simulink model "M1_ASE_be_SE"  (R2022b)
settings: Solver=ode4  StartTime=0.0  StopTime=200  FixedStep=1e-3  RelTol=1e-3  AbsTol=1e-3  EnableMultiTasking=on
values from neighbouring files (symbols this model uses):
  BAT = TWIZ.BAT    [init_M1_ASE_be_SE_main.m]
  CHAS = TWIZ.CHAS    [init_M1_ASE_be_SE_main.m]
  COR = TWIZ.COR    [init_M1_ASE_be_SE_main.m]
  ENV = TWIZ.ENV    [init_M1_ASE_be_SE_main.m]
  HACH = TWIZ.HACH    [init_M1_ASE_be_SE_main.m]
  MCC = TWIZ.MCC    [init_M1_ASE_be_SE_main.m]
  TRANS = TWIZ.TRANS    [init_M1_ASE_be_SE_main.m]
libraries: simulink x1
settings Model: Creator=Walter  LastModifiedBy=WENPAGNAGDE_JUSTIN
settings SolverCC: AutoScaleAbsTol=off  AlgebraicLoopSolver=TrustRegion
settings DataIOCC: LimitDataPoints=on  SaveFormat=Array  SignalLoggingSaveFormat=ModelDataLogs  ReturnWorkspaceOutputs=off
settings OptimizationCC: ExpressionDepthLimit=2147483647  InitFltsAndDblsToZero=on  LifeSpan=inf
settings DebuggingCC: UnderspecifiedInitializationDetection=Classic  MergeDetectMultiDrivingBlocksExec=none  SolverPrmCheckMsg=warning  FcnCallInpInsideContextMsg=warning  UnconnectedInputMsg=warning  UnconnectedOutputMsg=warning  UnconnectedLineMsg=warning  StateNameClashWarn=warning  SFUnexpectedBacktrackingDiag=warning  SFNoUnconditionalDefaultTransitionDiag=warning  SFExecutionAtInitializationDiag=none  SFMachineParentedDataDiag=warning  ArithmeticOperatorsInVariantConditions=warning
settings HardwareCC: ProdBitPerPointer=32  ProdBitPerSizeT=32  ProdBitPerPtrDiffT=32  ProdLargestAtomicFloat=None  ProdIntDivRoundTo=Undefined  ProdEndianess=Unspecified  ProdWordSize=32  ProdHWDeviceType=32-bit Generic
settings ModelReferenceCC: EnableRefExpFcnMdlSchedulingChecks=on  PropagateSignalLabelsOutOfModel=off
settings SFSimCC: SimUseLocalCustomCode=off  CustomCodeUndefinedFunction=UseInterfaceOnly
settings RTWCC: RTWUseLocalCustomCode=off  DLArmComputeVersion=19.05
settings CodeAppCC: StateflowObjectComments=on
settings GRTTargetCC: TargetLangStandard=C89/C90 (ANSI)  CombineOutputUpdateFcns=off  GRTInterface=on
settings ConfigComp: CovMetricSettings=dw  CovSaveCumulativeToWorkspaceVar=on  CovSaveSingleToWorkspaceVar=on

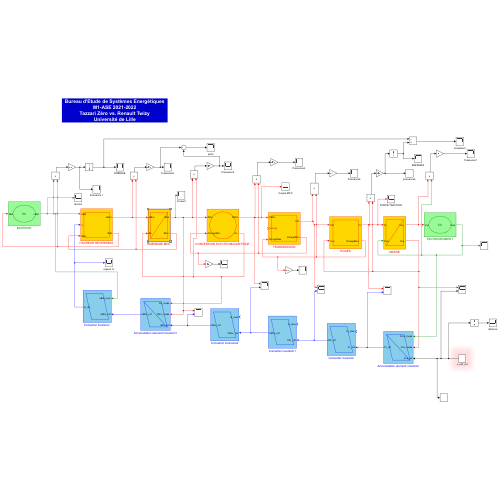
[thumbnail: Simulink's stored preview of the top-level diagram]
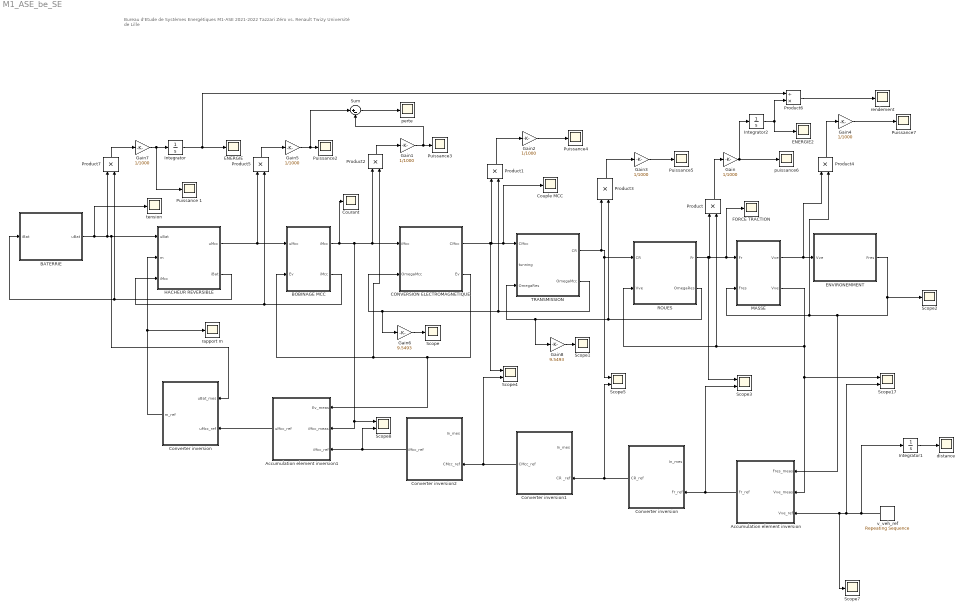
== system M1_ASE_be_SE ==
  note: Bureau d'Etude de Systèmes Energétiques
      | M1-ASE 2021-2022
      | Tazzari Zéro vs. Renault Twizy
      | Université de Lille
  Accumulation element inversion : Subsystem  AncestorBlock=simulink/SMC/Asservissement Correcteur IP
      settings: LibrarySourceBlock=|
      | simulink/SMC/Asservissement
      | Correcteur IP
      mask Display: plot(0,0,100,100, [10,30,90,70,10,90],[90,10,10,90,90,10])
  Accumulation element inversion1 : Subsystem  AncestorBlock=simulink/SMC/Asservissement Correcteur IP
      settings: LibrarySourceBlock=|
      | simulink/SMC/Asservissement
      | Correcteur IP
      mask Display: plot(0,0,100,100, [10,30,90,70,10,90],[90,10,10,90,90,10])
  BATERRIE : Subsystem  AncestorBlock=simulink/REM/SE
      settings: LibrarySourceBlock=simulink/REM/SE
      mask Display:
      | plot(0,0,100,100, 1.2*[50,57.68,60.77,63.08,64.97,66.58,68,69.26,70.4, 	71.42,72.36,78.28,80,78.28,72.36,71.42,70.4, 	69.26,68,66.58,64.97,63.08,60.77,57.68,50,42.32, 	39.23,36.92,35.03,33.42,32,30.74,29.6,28.58, 	27.64,21.72,20,21.72,27.64,28.58,29.6,30.74,32, 	33.42,35.03,36.92,39.23,42.32,50]-10, 1.2*[20,21,22,23,24,25,26,27,28,29,30,40,50,60,70,71,72, 	73,74,75,76,77,78,79,80,79,78,77,76,75,74,73,72, 	71,70,60,50,40,30,29,28,27,26,25,24,23,22,21,20]-10)
      | disp('ES')
  BOBINAGE MCC : Subsystem  AncestorBlock=simulink/REM/EA  mask(CM){}
      settings: LibrarySourceBlock=simulink/REM/EA
      mask Display: plot(0,0,100,100,[10,10,90,90,10],[90,10,10,90,90], [10,90],[10,90])
  "CONVERSION ELECTROMAGNETIQUE " : Subsystem  AncestorBlock=simulink/REM/EC EM
      settings: LibrarySourceBlock=simulink/REM/EC EM
      mask Display: plot(0,0,100,100, 1.4*[50,57.68,60.77,63.08,64.97,66.58,68,69.26,70.4, 	71.42,72.36,78.28,80,78.28,72.36,71.42,70.4, 	69.26,68,66.58,64.97,63.08,60.77,57.68,50,42.32, 	39.23,36.92,35.03,33.42,32,30.74,29.6,28.58, 	27.64,21.72,20,21.72,27.64,28.58,29.6,30.74,32, 	33.42,35.03,36.92,39.23,42.32,50]-20, 1.4*[20,21,22,23,24,25,26,27,28,29,30,40,50,60,70,71,72, 	73,74,75,76,77,78,79,80,79,78,77,76,75,74,73,72, 	71,70,60,50,40,30,29,28,27,26,25,24,23,22,21,20]-20)
  Converter inversion : Subsystem  AncestorBlock=simulink/SMC/Inversion EC avec mesure
      settings: LibrarySourceBlock=|
      | simulink/SMC/Inversion EC
      | avec mesure
      mask Display: plot(0,0,100,100,[10,30,90,70,10],[90,10,10,90,90])
  "Converter inversion " : Subsystem  AncestorBlock=simulink/SMC/Inversion EC avec mesure
      settings: LibrarySourceBlock=|
      | simulink/SMC/Inversion EC
      | avec mesure
      mask Display: plot(0,0,100,100,[10,30,90,70,10],[90,10,10,90,90])
  Converter inversion1 : Subsystem  AncestorBlock=simulink/SMC/Inversion EC avec mesure
      settings: LibrarySourceBlock=|
      | simulink/SMC/Inversion EC
      | avec mesure
      mask Display: plot(0,0,100,100,[10,30,90,70,10],[90,10,10,90,90])
  Converter inversion2 : Subsystem  AncestorBlock=simulink/SMC/Inversion EC avec mesure
      settings: LibrarySourceBlock=|
      | simulink/SMC/Inversion EC
      | avec mesure
      mask Display: plot(0,0,100,100,[10,30,90,70,10],[90,10,10,90,90])
  Couple MCC : Scope
  Courant : Scope
  ENERGIE : Scope
  ENERGIE2 : Scope
  ENVIRONEMMENT : Subsystem  AncestorBlock=simulink/REM/SE
      settings: LibrarySourceBlock=simulink/REM/SE
      mask Display:
      | plot(0,0,100,100, 1.2*[50,57.68,60.77,63.08,64.97,66.58,68,69.26,70.4, 	71.42,72.36,78.28,80,78.28,72.36,71.42,70.4, 	69.26,68,66.58,64.97,63.08,60.77,57.68,50,42.32, 	39.23,36.92,35.03,33.42,32,30.74,29.6,28.58, 	27.64,21.72,20,21.72,27.64,28.58,29.6,30.74,32, 	33.42,35.03,36.92,39.23,42.32,50]-10, 1.2*[20,21,22,23,24,25,26,27,28,29,30,40,50,60,70,71,72, 	73,74,75,76,77,78,79,80,79,78,77,76,75,74,73,72, 	71,70,60,50,40,30,29,28,27,26,25,24,23,22,21,20]-10)
      | disp('ES')
  FORCE TRACTION : Scope
  Gain{,1..5,7} (7 alike) : Gain  Gain=1/1000
  Gain6 : Gain  Gain=9.5493
  Gain8 : Gain  Gain=9.5493
  HACHEUR REVERSIBLE : Subsystem  AncestorBlock=simulink/REM/EC Elec  mask(Hacheur){}
      settings: LibrarySourceBlock=simulink/REM/EC Elec
      mask Display: plot(0,0,100,100,[10,10,90,90,10],[90,10,10,90,90])
  Integrator : Integrator
  Integrator1 : Integrator
  Integrator2 : Integrator
  MASSE : Subsystem  AncestorBlock=simulink/REM/EA  mask(CM){}
      settings: LibrarySourceBlock=simulink/REM/EA
      mask Display: plot(0,0,100,100,[10,10,90,90,10],[90,10,10,90,90], [10,90],[10,90])
  Product{,1..5,7} (7 alike) : Product
  Product6 : Product  Inputs=/*
  Puissance 1 : Scope
  Puissance{2..5,7} (5 alike) : Scope
  ROUES : Subsystem  AncestorBlock=simulink/REM/EC Elec  mask(Hacheur){}
      settings: LibrarySourceBlock=simulink/REM/EC Elec
      mask Display: plot(0,0,100,100,[10,10,90,90,10],[90,10,10,90,90])
  Scope{,1..2,7} (4 alike) : Scope
  Scope{3..5,8,17} (5 alike) : Scope  NumInputPorts=2
  Sum : Sum  Inputs=|+-
  TRANSMISSION : Subsystem  AncestorBlock=simulink/REM/EC Elec  mask(Hacheur){}
      settings: LibrarySourceBlock=simulink/REM/EC Elec
      mask Display: plot(0,0,100,100,[10,10,90,90,10],[90,10,10,90,90])
  distance : Scope
  perte : Scope
  puissance6 : Scope
  rapport m : Scope
  rendement : Scope
  tension : Scope
  v_veh_ref : simulink/Sources/Repeating Sequence  rep_seq_t=CYCL.time_ECE  rep_seq_y=CYCL.velocity_ECE
  wires:
  "Converter inversion "/1(m_ref) -> rapport m/1, HACHEUR REVERSIBLE/2(m)
  BATERRIE/1("uBat ") -> tension/1, Product7/1, "Converter inversion "/1(uBat_mes), HACHEUR REVERSIBLE/1(uBat)
  MASSE/2("Vve ") -> Product/2, ROUES/2(Vve), Accumulation element inversion/2(Vve_meas), Scope17/1
  Accumulation element inversion/1(Fr_ref) -> Scope3/2, Converter inversion/2(Fr_ref)
  ROUES/1(Fr) -> FORCE TRACTION/1, MASSE/1(Fr), Product/1, Scope3/1
  Converter inversion/1(CR_ref) -> Scope5/2, Converter inversion1/2(CR _ref)
  TRANSMISSION/1("CR ") -> Scope5/1, ROUES/1("CR  "), Product3/1
  Converter inversion1/1(CMcc_ref) -> Scope4/2, Converter inversion2/2(CMcc_ref)
  TRANSMISSION/2(OmegaMcc) -> Gain6/1, "CONVERSION ELECTROMAGNETIQUE "/2(OmegaMcc), Product1/2
  BOBINAGE MCC/1(iMcc) -> Courant/1, Product2/1, "CONVERSION ELECTROMAGNETIQUE "/1(iMcc), Scope8/1, Accumulation element inversion1/2(iMcc_meas)
  BOBINAGE MCC/2("iMcc ") -> Product5/2, HACHEUR REVERSIBLE/3(iMcc)
  Converter inversion2/1(iMcc_ref) -> Scope8/2, Accumulation element inversion1/3(iMcc_ref)
  "CONVERSION ELECTROMAGNETIQUE "/2("Ev ") -> Product2/2, BOBINAGE MCC/2(Ev), Accumulation element inversion1/1(Ev_meas)
  Product2/1 -> Gain1/1
  Product1/1 -> Gain2/1
  Product/1 -> Gain/1
  Gain1/1 -> Puissance3/1, Sum/2
  Gain2/1 -> Puissance4/1
  Gain3/1 -> Puissance5/1
  MASSE/1("Vve  ") -> Product4/1, ENVIRONEMMENT/1(Vve)
  ENVIRONEMMENT/1(Fres) -> Scope2/1, Accumulation element inversion/1(Fres_meas), Product4/2, MASSE/2(Fres)
  HACHEUR REVERSIBLE/2(iBat) -> Product7/2, BATERRIE/1(iBat)
  Accumulation element inversion1/1(uMcc_ref) -> "Converter inversion "/2(uMcc_ref)
  HACHEUR REVERSIBLE/1(uMcc) -> Product5/1, BOBINAGE MCC/1(uMcc)
  Gain5/1 -> Sum/1, Puissance2/1
  Product5/1 -> Gain5/1
  Product7/1 -> Gain7/1
  Product3/1 -> Gain3/1
  Integrator/1 -> Product6/1, ENERGIE/1
  Gain7/1 -> Puissance 1/1, Integrator/1
  v_veh_ref/1 -> Integrator1/1, Scope17/2, Scope7/1, Accumulation element inversion/3("\t\tVve_ref")
  Integrator1/1 -> distance/1
  Sum/1 -> perte/1
  Product6/1 -> rendement/1
  Gain/1 -> puissance6/1, Integrator2/1
  Product4/1 -> Gain4/1
  Integrator2/1 -> ENERGIE2/1, Product6/2
  Gain4/1 -> Puissance7/1
  Gain6/1 -> Scope/1
  Gain8/1 -> Scope1/1
  ROUES/2("OmegaRes   ") -> Product3/2, Gain8/1, TRANSMISSION/3("OmegaRes ")
  "CONVERSION ELECTROMAGNETIQUE "/1(CMcc) -> TRANSMISSION/1("CMcc "), Couple MCC/1, Product1/1, Scope4/1

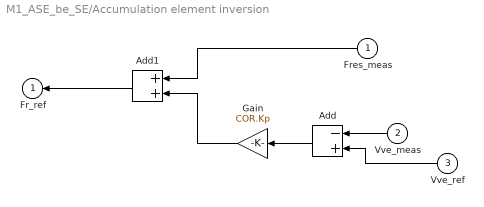
== system M1_ASE_be_SE/Accumulation element inversion ==
  Fres_meas : Inport
  Vve_meas : Inport  Port=2
  "\t\tVve_ref" : Inport  Port=3
  Add : Sum  Inputs=-+
  Add1 : Sum
  Gain : Gain  Gain=COR.Kp
  Fr_ref : Outport  InitialOutput=0
  wires:
  "\t\tVve_ref"/1 -> Add/2
  Vve_meas/1 -> Add/1
  Fres_meas/1 -> Add1/1
  Add/1 -> Gain/1
  Gain/1 -> Add1/2
  Add1/1 -> Fr_ref/1

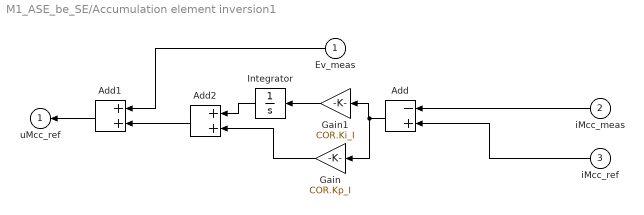
== system M1_ASE_be_SE/Accumulation element inversion1 ==
  Ev_meas : Inport
  iMcc_meas : Inport  Port=2
  iMcc_ref : Inport  Port=3
  Add : Sum  Inputs=-+
  Add1 : Sum
  Add2 : Sum
  Gain : Gain  Gain=COR.Kp_I
  Gain1 : Gain  Gain=COR.Ki_I
  Integrator : Integrator
  uMcc_ref : Outport  InitialOutput=0
  wires:
  iMcc_meas/1 -> Add/1
  iMcc_ref/1 -> Add/2
  Ev_meas/1 -> Add1/1
  Add1/1 -> uMcc_ref/1
  Add/1 -> Gain/1, Gain1/1
  Gain/1 -> Add2/2
  Gain1/1 -> Integrator/1
  Integrator/1 -> Add2/1
  Add2/1 -> Add1/2

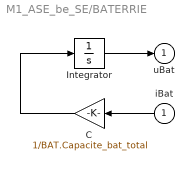
== system M1_ASE_be_SE/BATERRIE ==
  iBat : Inport
  C : Gain  Gain=1/BAT.Capacite_bat_total
  Integrator : Integrator  InitialCondition=100.8
  "uBat " : Outport  InitialOutput=0
  wires:
  Integrator/1 -> "uBat "/1
  iBat/1 -> C/1
  C/1 -> Integrator/1

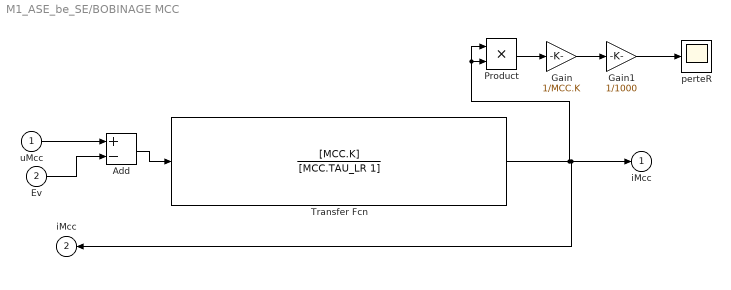
== system M1_ASE_be_SE/BOBINAGE MCC ==
  uMcc : Inport
  Ev : Inport  Port=2
  Add : Sum  Inputs=+-
  Gain : Gain  Gain=1/MCC.K
  Gain1 : Gain  Gain=1/1000
  Product : Product
  Transfer Fcn : TransferFcn  Numerator=[MCC.K]  Denominator=[MCC.TAU_LR 1]
  perteR : Scope
  iMcc : Outport  InitialOutput=0
  "iMcc " : Outport  Port=2  InitialOutput=0
  wires:
  uMcc/1 -> Add/1
  Ev/1 -> Add/2
  Add/1 -> Transfer Fcn/1
  Transfer Fcn/1 -> "iMcc "/1, iMcc/1, Product/1, Product/2
  Product/1 -> Gain/1
  Gain/1 -> Gain1/1
  Gain1/1 -> perteR/1

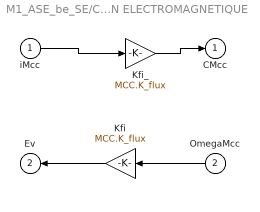
== system M1_ASE_be_SE/CONVERSION ELECTROMAGNETIQUE  ==
  iMcc : Inport
  OmegaMcc : Inport  Port=2
  Kfi : Gain  Gain=MCC.K_flux
  Kfi_ : Gain  Gain=MCC.K_flux
  CMcc : Outport  InitialOutput=0
  "Ev " : Outport  Port=2  InitialOutput=0
  wires:
  iMcc/1 -> Kfi_/1
  Kfi_/1 -> CMcc/1
  Kfi/1 -> "Ev "/1
  OmegaMcc/1 -> Kfi/1

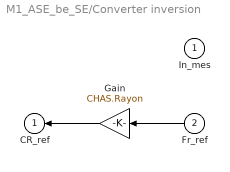
== system M1_ASE_be_SE/Converter inversion ==
  In_mes : Inport
  Fr_ref : Inport  Port=2
  Gain : Gain  Gain=CHAS.Rayon
  CR_ref : Outport  InitialOutput=0
  wires:
  Fr_ref/1 -> Gain/1
  Gain/1 -> CR_ref/1

== system M1_ASE_be_SE/Converter inversion  ==
  uBat_mes : Inport
  uMcc_ref : Inport  Port=2
  Product : Product  Inputs=/*
  m_ref : Outport  InitialOutput=0
  wires:
  uMcc_ref/1 -> Product/2
  uBat_mes/1 -> Product/1
  Product/1 -> m_ref/1

== system M1_ASE_be_SE/Converter inversion1 ==
  In_mes : Inport
  CR _ref : Inport  Port=2
  Gain : Gain  Gain=1/TRANS.k_red
  CMcc_ref : Outport  InitialOutput=0
  wires:
  Gain/1 -> CMcc_ref/1
  CR _ref/1 -> Gain/1

== system M1_ASE_be_SE/Converter inversion2 ==
  In_mes : Inport
  CMcc_ref : Inport  Port=2
  Kfi : Gain  Gain=1/MCC.K_flux
  iMcc_ref : Outport  InitialOutput=0
  wires:
  Kfi/1 -> iMcc_ref/1
  CMcc_ref/1 -> Kfi/1

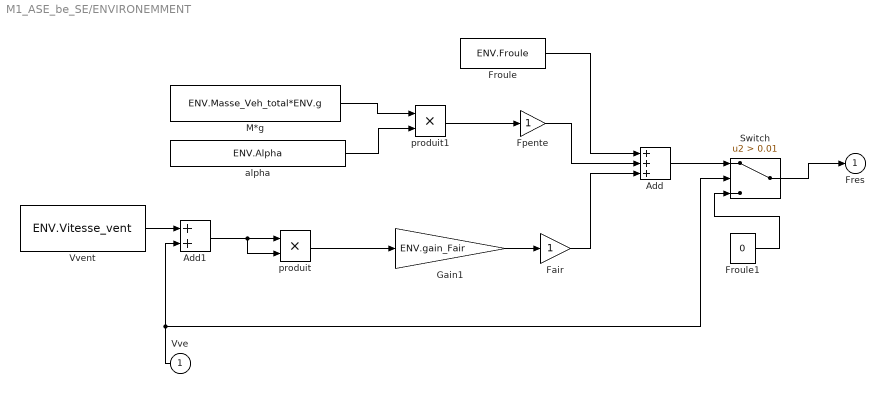
== system M1_ASE_be_SE/ENVIRONEMMENT ==
  Vve : Inport
  Add : Sum  Inputs=+++
  Add1 : Sum
  Fair : Gain
  Fpente : Gain
  Froule : Constant  Value=ENV.Froule
  Froule1 : Constant  Value=0
  Gain1 : Gain  Gain=ENV.gain_Fair
  M*g : Constant  Value=ENV.Masse_Veh_total*ENV.g
  Switch : Switch  Criteria=u2 > Threshold  Threshold=0.01  SaturateOnIntegerOverflow=off  InputSameDT=off
  Vvent : Constant  Value=ENV.Vitesse_vent
  alpha : Constant  Value=ENV.Alpha
  produit : Product  Inputs=**
  produit1 : Product  Inputs=**
  Fres : Outport  InitialOutput=0
  wires:
  Froule/1 -> Add/1
  Vvent/1 -> Add1/1
  Add1/1 -> produit/2, produit/1
  produit/1 -> Gain1/1
  M*g/1 -> produit1/1
  alpha/1 -> produit1/2
  produit1/1 -> Fpente/1
  Fpente/1 -> Add/2
  Fair/1 -> Add/3
  Gain1/1 -> Fair/1
  Vve/1 -> Switch/2, Add1/2
  Add/1 -> Switch/1
  Switch/1 -> Fres/1
  Froule1/1 -> Switch/3

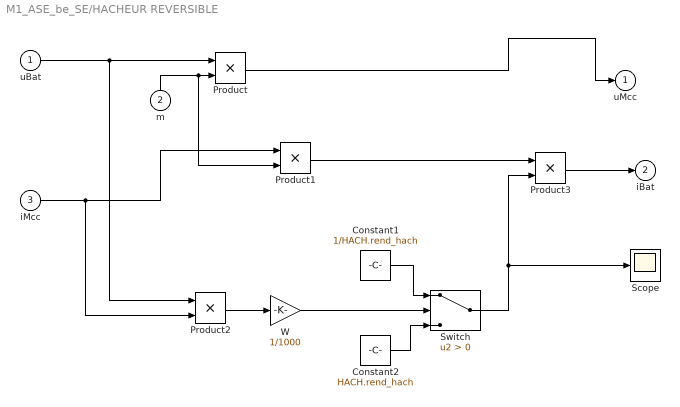
== system M1_ASE_be_SE/HACHEUR REVERSIBLE ==
  uBat : Inport
  m : Inport  Port=2
  iMcc : Inport  Port=3
  Constant1 : Constant  Value=1/HACH.rend_hach
  Constant2 : Constant  Value=HACH.rend_hach
  Product{,1..3} (4 alike) : Product
  Scope : Scope
  Switch : Switch  Criteria=u2 > Threshold  SaturateOnIntegerOverflow=off  InputSameDT=off
  W : Gain  Gain=1/1000
  uMcc : Outport  InitialOutput=0
  iBat : Outport  Port=2  InitialOutput=0
  wires:
  uBat/1 -> Product2/1, Product/1
  m/1 -> Product1/2, Product/2
  iMcc/1 -> Product2/2, Product1/1
  Constant1/1 -> Switch/1
  Constant2/1 -> Switch/3
  Product2/1 -> W/1
  W/1 -> Switch/2
  Product/1 -> uMcc/1
  Product1/1 -> Product3/1
  Switch/1 -> Scope/1, Product3/2
  Product3/1 -> iBat/1

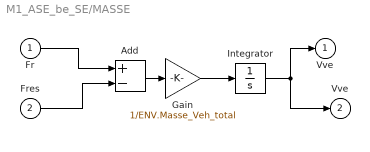
== system M1_ASE_be_SE/MASSE ==
  Fr : Inport
  Fres : Inport  Port=2
  Add : Sum  Inputs=+-
  Gain : Gain  Gain=1/ENV.Masse_Veh_total
  Integrator : Integrator
  "Vve  " : Outport  InitialOutput=0
  "Vve " : Outport  Port=2  InitialOutput=0
  wires:
  Fr/1 -> Add/1
  Fres/1 -> Add/2
  Add/1 -> Gain/1
  Gain/1 -> Integrator/1
  Integrator/1 -> "Vve "/1, "Vve  "/1

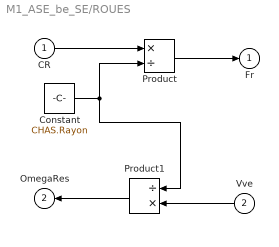
== system M1_ASE_be_SE/ROUES ==
  "CR  " : Inport
  Vve : Inport  Port=2
  Constant : Constant  Value=CHAS.Rayon
  Product : Product  Inputs=*/
  Product1 : Product  Inputs=/*
  Fr : Outport  InitialOutput=0
  "OmegaRes   " : Outport  Port=2  InitialOutput=0
  wires:
  "CR  "/1 -> Product/1
  Product/1 -> Fr/1
  Constant/1 -> Product1/1, Product/2
  Vve/1 -> Product1/2
  Product1/1 -> "OmegaRes   "/1

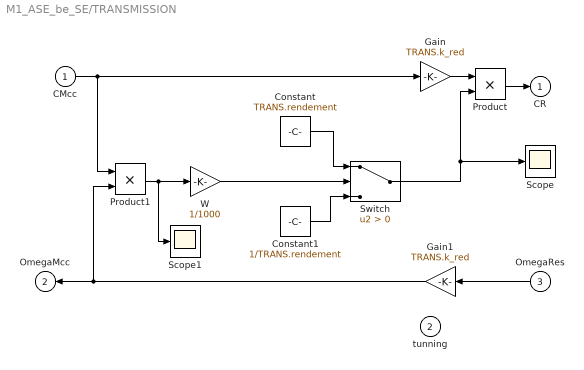
== system M1_ASE_be_SE/TRANSMISSION ==
  "CMcc " : Inport
  tunning : Inport  Port=2
  "OmegaRes " : Inport  Port=3
  Constant : Constant  Value=TRANS.rendement
  Constant1 : Constant  Value=1/TRANS.rendement
  Gain : Gain  Gain=TRANS.k_red
  Gain1 : Gain  Gain=TRANS.k_red
  Product : Product
  Product1 : Product
  Scope : Scope
  Scope1 : Scope
  Switch : Switch  Criteria=u2 > Threshold  SaturateOnIntegerOverflow=off  InputSameDT=off
  W : Gain  Gain=1/1000
  "CR " : Outport  InitialOutput=0
  OmegaMcc : Outport  Port=2  InitialOutput=0
  wires:
  Gain1/1 -> Product1/2, OmegaMcc/1
  "OmegaRes "/1 -> Gain1/1
  "CMcc "/1 -> Product1/1, Gain/1
  Gain/1 -> Product/1
  Product1/1 -> Scope1/1, W/1
  W/1 -> Switch/2
  Constant/1 -> Switch/1
  Constant1/1 -> Switch/3
  Switch/1 -> Scope/1, Product/2
  Product/1 -> "CR "/1
